simulink model "FinalSim"  (R2022b)
settings: Solver=VariableStepAuto  StartTime=0.0  StopTime=10  RelTol=1e-3
libraries: eeGeneralControl x3
(part 1 of 7)
settings Model: Creator=Dhruv  LastModifiedBy=Dhruv

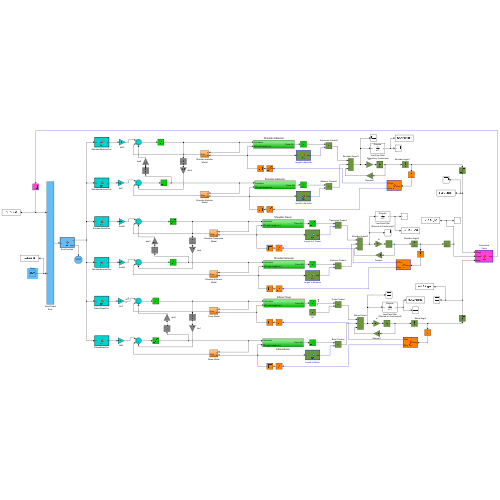
[thumbnail: Simulink's stored preview of the top-level diagram]
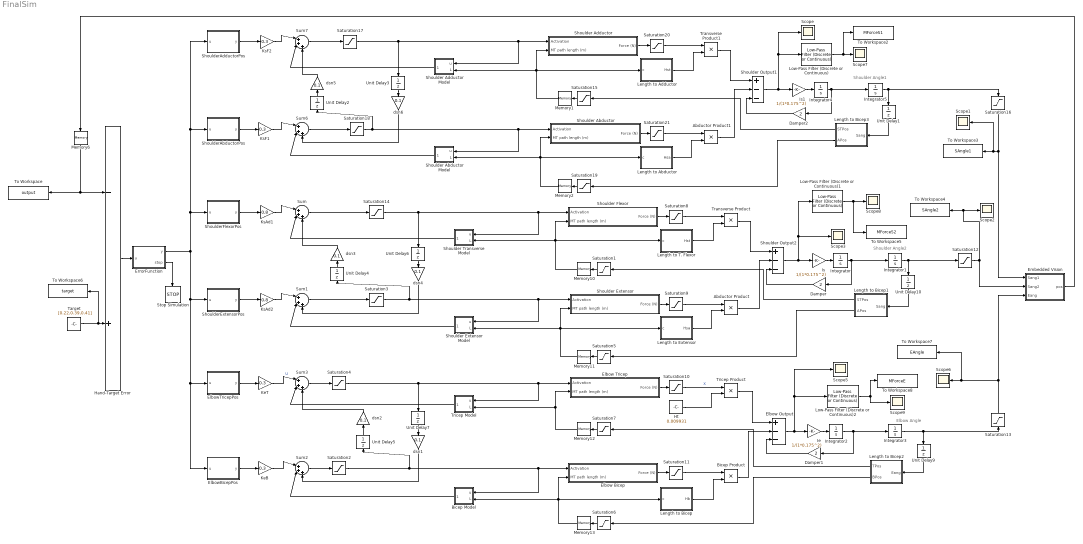
== system FinalSim ==
  note: Shoulder Angle2
  note: Elbow Angle
  note: Shoulder Angle1
  Abductor Product : Product  RndMeth=Zero
  Abductor Product1 : Product  RndMeth=Zero
  Bicep Model : Subsystem
  Bicep Product : Product  RndMeth=Zero
  Damper : Gain  Gain=2
  Damper1 : Gain  Gain=2
  Damper2 : Gain  Gain=2
  Elbow Bicep : Subsystem
  Elbow Output : Sum  Inputs=+--
  Elbow Tricep : Subsystem
  "ElbowBicepPos " : MATLAB Function  TreatAsAtomicUnit=on
  "ElbowTricepPos " : MATLAB Function  TreatAsAtomicUnit=on
  Embedded Vision : MATLAB Function  TreatAsAtomicUnit=on
  ErrorFunction : MATLAB Function  TreatAsAtomicUnit=on
  Hand-Target Error : Sum  Inputs=-+
  Ht : Constant  Value=0.009931  VectorParams1D=off
  Ie : Gain  Gain=1/(1*0.175^2)
  Integrator : Integrator  ZeroCross=off
  Integrator1 : Integrator  InitialCondition=0.5673
  Integrator2 : Integrator  ZeroCross=off
  Integrator3 : Integrator  InitialCondition=0.2362
  Integrator4 : Integrator  ZeroCross=off
  Integrator5 : Integrator  InitialCondition=0.838
  Is : Gain  Gain=1/(1*0.175^2)
  Is1 : Gain  Gain=1/(1*0.175^2)
  KeB : Gain  Gain=0.3
  KeT : Gain  Gain=0.3
  KsAd1 : Gain  Gain=0.8
  KsAd2 : Gain  Gain=0.8
  KsF1 : Gain  Gain=0.3
  KsF2 : Gain  Gain=0.3
  Length to Abductor : MATLAB Function  TreatAsAtomicUnit=on
  Length to Adductor : MATLAB Function  TreatAsAtomicUnit=on
  Length to Bicep : MATLAB Function  TreatAsAtomicUnit=on
  Length to Bicep1 : MATLAB Function  TreatAsAtomicUnit=on
  Length to Bicep2 : MATLAB Function  TreatAsAtomicUnit=on
  Length to Bicep3 : MATLAB Function  TreatAsAtomicUnit=on
  Length to Extensor : MATLAB Function  TreatAsAtomicUnit=on
  Length to T. Flexor : MATLAB Function  TreatAsAtomicUnit=on
  Low-Pass Filter (Discrete or Continuous) : eeGeneralControl/Low-Pass Filter (Discrete or Continuous)  K=1  T=1  B=inf  A=-inf  init_option=Inherited from block input  x0=0  Ts=-1
  Low-Pass Filter (Discrete or Continuous)1 : eeGeneralControl/Low-Pass Filter (Discrete or Continuous)  K=1  T=1  B=inf  A=-inf  init_option=Inherited from block input  x0=0  Ts=-1
  Low-Pass Filter (Discrete or Continuous)2 : eeGeneralControl/Low-Pass Filter (Discrete or Continuous)  K=1  T=1  B=inf  A=-inf  init_option=Inherited from block input  x0=0  Ts=-1
  Memory1 : Memory  InitialCondition=0.08165  InheritSampleTime=on
  Memory10 : Memory  InitialCondition=0.08943  InheritSampleTime=on
  Memory11 : Memory  InitialCondition=0.06893  InheritSampleTime=on
  Memory12 : Memory  InitialCondition=0.1729  InheritSampleTime=on
  Memory13 : Memory  InitialCondition=0.1076  InheritSampleTime=on
  Memory2 : Memory  InitialCondition=0.06454  InheritSampleTime=on
  Memory6 : Memory  InitialCondition=[0.16960,0.1895620 , 0.2307203]  InheritSampleTime=on
  Saturation1 : Saturate  UpperLimit=0.095  LowerLimit=0.068  LinearizeAsGain=off
  Saturation{8..11,20..21} (6 alike) : Saturate  UpperLimit=200  LowerLimit=0  LinearizeAsGain=off
  Saturation12 : Saturate  UpperLimit=3.14159  LowerLimit=-1.0472  LinearizeAsGain=off
  Saturation13 : Saturate  UpperLimit=2.61799  LowerLimit=0  LinearizeAsGain=off
  Saturation{2..4,14,17..18} (6 alike) : Saturate  UpperLimit=1  LowerLimit=0  LinearizeAsGain=off
  Saturation15 : Saturate  UpperLimit=0.095  LowerLimit=0.068  LinearizeAsGain=off
  Saturation16 : Saturate  UpperLimit=2.61799  LowerLimit=-0.872665  LinearizeAsGain=off
  Saturation19 : Saturate  UpperLimit=0.075  LowerLimit=0.057  LinearizeAsGain=off
  Saturation5 : Saturate  UpperLimit=0.075  LowerLimit=0.057  LinearizeAsGain=off
  Saturation6 : Saturate  UpperLimit=0.15  LowerLimit=0.1  LinearizeAsGain=off  RndMeth=Nearest
  Saturation7 : Saturate  UpperLimit=0.17  LowerLimit=0.1  LinearizeAsGain=off
  Scope{,1..3,5..9} (9 alike) : Scope
  Shoulder Abductor : Subsystem
  Shoulder Abductor Model : Subsystem
  Shoulder Adductor : Subsystem
  Shoulder Adductor Model : Subsystem
  Shoulder Extensor : Subsystem
  Shoulder Extensor Model : Subsystem
  Shoulder Flexor : Subsystem
  Shoulder Output1 : Sum  Inputs=+--
  Shoulder Output2 : Sum  Inputs=+--
  Shoulder Transverse Model : Subsystem
  "ShoulderAbductorPos " : MATLAB Function  TreatAsAtomicUnit=on
  "ShoulderAdductorPos " : MATLAB Function  TreatAsAtomicUnit=on
  "ShoulderExtensorPos " : MATLAB Function  TreatAsAtomicUnit=on
  "ShoulderFlexorPos " : MATLAB Function  TreatAsAtomicUnit=on
  Stop Simulation : Stop
  Sum{,1..3,6..7} (6 alike) : Sum  Inputs=|+++  OutMin=[-10]  OutMax=[10]  SampleTime=0.04
  Target : Constant  Value=[0.22,0.39,0.41]  VectorParams1D=off
  To Workspace : ToWorkspace  VariableName=output  SaveFormat=Timeseries  SampleTime=-1
  To Workspace2 : ToWorkspace  VariableName=MForceS1  SaveFormat=Timeseries  SampleTime=-1
  To Workspace3 : ToWorkspace  VariableName=SAngle1  SaveFormat=Timeseries  SampleTime=-1
  To Workspace4 : ToWorkspace  VariableName=SAngle2  SaveFormat=Timeseries  SampleTime=-1
  To Workspace5 : ToWorkspace  VariableName=MForceS2  SaveFormat=Timeseries  SampleTime=-1
  To Workspace6 : ToWorkspace  VariableName=target  SaveFormat=Timeseries  SampleTime=-1
  To Workspace7 : ToWorkspace  VariableName=EAngle  SaveFormat=Timeseries  SampleTime=-1
  To Workspace8 : ToWorkspace  VariableName=MForceE  SaveFormat=Timeseries  SampleTime=-1
  Transverse Product : Product  RndMeth=Zero
  Transverse Product1 : Product  RndMeth=Zero
  Tricep Model : Subsystem
  Tricep Product : Product  RndMeth=Zero
  Unit Delay{1..7,9..10} (9 alike) : UnitDelay  SampleTime=-1
  dsn{1..6} (6 alike) : Gain  Gain=0.1
  wires:
  Shoulder Transverse Model/1(Fom) -> Sum/2
  Is/1 -> Integrator/1
  Ie/1 -> Integrator2/1
  Memory10/1 -> Shoulder Flexor/2(MT path length (m)), Length to T. Flexor/1(c), Shoulder Transverse Model/2(L)
  Saturation13/1 -> Embedded Vision/3(Eang), To Workspace7/1, Scope6/1
  Unit Delay5/1 -> dsn2/1
  Integrator1/1 -> Unit Delay10/1, Saturation12/1
  Saturation3/1 -> Unit Delay4/1, Shoulder Extensor Model/1(u), Shoulder Extensor/1(Activation)
  Damper/1 -> Shoulder Output2/3
  dsn3/1 -> Sum/3
  Saturation11/1 -> Bicep Product/1
  Saturation6/1 -> Memory13/1
  Target/1 -> To Workspace6/1, Hand-Target Error/2
  Damper1/1 -> Elbow Output/3
  Saturation8/1 -> Transverse Product/1
  Saturation10/1 -> Tricep Product/1  "X"
  Saturation9/1 -> Abductor Product/1
  Elbow Tricep/1(Force (N)) -> Saturation10/1
  Memory11/1 -> Shoulder Extensor/2(MT path length (m)), Length to Extensor/1(c), Shoulder Extensor Model/2(L)
  Memory13/1 -> Length to Bicep/1(c), Bicep Model/2(L), Elbow Bicep/2(MT path length (m))
  Integrator/1 -> Damper/1, Integrator1/1
  Saturation12/1 -> To Workspace4/1, Scope2/1, Embedded Vision/2(Sang2)
  Transverse Product/1 -> Shoulder Output2/1
  Abductor Product/1 -> Shoulder Output2/2
  Length to T. Flexor/1(Hst) -> Transverse Product/2
  Length to Extensor/1(Hsa) -> Abductor Product/2
  Memory12/1 -> Elbow Tricep/2(MT path length (m)), Tricep Model/2(L)
  Saturation7/1 -> Memory12/1
  Shoulder Flexor/1(Force (N)) -> Saturation8/1
  Tricep Product/1 -> Elbow Output/1
  Ht/1 -> Tricep Product/2
  Elbow Bicep/1(Force (N)) -> Saturation11/1
  Integrator3/1 -> Saturation13/1, Unit Delay9/1
  Unit Delay7/1 -> dsn1/1
  Integrator2/1 -> Damper1/1, Integrator3/1
  Saturation1/1 -> Memory10/1
  Length to Bicep/1(Hb) -> Bicep Product/2
  dsn1/1 -> Sum2/3
  Memory6/1 -> To Workspace/1, Hand-Target Error/1
  Unit Delay4/1 -> dsn3/1
  Unit Delay6/1 -> dsn4/1
  Shoulder Extensor/1(Force (N)) -> Saturation9/1
  Saturation5/1 -> Memory11/1
  Sum/1 -> Saturation14/1
  Bicep Product/1 -> Elbow Output/2
  Shoulder Abductor/1(Force (N)) -> Saturation21/1
  Unit Delay3/1 -> dsn6/1
  Saturation19/1 -> Memory2/1
  Unit Delay2/1 -> dsn5/1
  Saturation15/1 -> Memory1/1
  Shoulder Output1/1 -> Is1/1, Scope/1, Low-Pass Filter (Discrete or Continuous)/1
  Shoulder Adductor/1(Force (N)) -> Saturation20/1
  Abductor Product1/1 -> Shoulder Output1/2
  Saturation16/1 -> Embedded Vision/1(Sang1), Scope1/1, To Workspace3/1
  Integrator4/1 -> Damper2/1, Integrator5/1
  Length to Abductor/1(Hsa) -> Abductor Product1/2
  Damper2/1 -> Shoulder Output1/3
  Memory2/1 -> Shoulder Abductor/2(MT path length (m)), Length to Abductor/1(c), Shoulder Abductor Model/2(L)
  Length to Adductor/1(Hst) -> Transverse Product1/2
  Is1/1 -> Integrator4/1
  Transverse Product1/1 -> Shoulder Output1/1
  Memory1/1 -> Shoulder Adductor/2(MT path length (m)), Length to Adductor/1(c), Shoulder Adductor Model/2(L)
  Saturation20/1 -> Transverse Product1/1
  Saturation21/1 -> Abductor Product1/1
  Hand-Target Error/1 -> ErrorFunction/1(u)
  "ShoulderFlexorPos "/1(y) -> KsAd1/1
  "ShoulderExtensorPos "/1(y) -> KsAd2/1
  "ElbowTricepPos "/1(y) -> KeT/1
  "ElbowBicepPos "/1(y) -> KeB/1
  "ShoulderAbductorPos "/1(y) -> KsF1/1
  "ShoulderAdductorPos "/1(y) -> KsF2/1
  ErrorFunction/2(stop) -> Stop Simulation/1
  Embedded Vision/1(pos) -> Memory6/1
  Integrator5/1 -> Saturation16/1, Unit Delay1/1
  Unit Delay9/1 -> Length to Bicep2/1(Eang)
  Length to Bicep2/1(TPos) -> Saturation7/1
  Length to Bicep2/2(BPos) -> Saturation6/1
  Sum3/1 -> Saturation4/1
  dsn2/1 -> Sum3/3
  Tricep Model/1(Fom) -> Sum3/2
  dsn4/1 -> Sum1/3
  Shoulder Extensor Model/1(Fom) -> Sum1/2
  Sum2/1 -> Saturation2/1
  Bicep Model/1(Fom) -> Sum2/2
  Sum6/1 -> Saturation18/1
  Sum7/1 -> Saturation17/1
  dsn5/1 -> Sum7/3
  Shoulder Adductor Model/1(Fom) -> Sum7/2
  dsn6/1 -> Sum6/3
  Shoulder Abductor Model/1(Fom) -> Sum6/2
  Low-Pass Filter (Discrete or Continuous)/1 -> Scope7/1, To Workspace2/1
  Low-Pass Filter (Discrete or Continuous)1/1 -> To Workspace5/1, Scope8/1
  Shoulder Output2/1 -> Low-Pass Filter (Discrete or Continuous)1/1, Scope3/1, Is/1
  Low-Pass Filter (Discrete or Continuous)2/1 -> Scope9/1, To Workspace8/1
  Elbow Output/1 -> Scope5/1, Low-Pass Filter (Discrete or Continuous)2/1, Ie/1
  Unit Delay1/1 -> Length to Bicep3/1(Sang)
  Unit Delay10/1 -> Length to Bicep1/1(Sang)
  Length to Bicep1/2(APos) -> Saturation5/1
  Length to Bicep1/1(STPos) -> Saturation1/1
  ErrorFunction/1(y) -> "ShoulderAdductorPos "/1(u), "ShoulderAbductorPos "/1(u), "ShoulderFlexorPos "/1(u), "ElbowBicepPos "/1(u), "ElbowTricepPos "/1(u), "ShoulderExtensorPos "/1(u)
  Length to Bicep3/2(APos) -> Saturation19/1
  Length to Bicep3/1(STPos) -> Saturation15/1
  KsAd1/1 -> Sum/1
  KsAd2/1 -> Sum1/1
  KeB/1 -> Sum2/1
  KeT/1 -> Sum3/1  "U"
  Saturation4/1 -> Unit Delay7/1, Tricep Model/1(u), Elbow Tricep/1(Activation)
  Saturation2/1 -> Unit Delay5/1, Bicep Model/1(u), Elbow Bicep/1(Activation)
  Sum1/1 -> Saturation3/1
  Saturation14/1 -> Unit Delay6/1, Shoulder Transverse Model/1(u), Shoulder Flexor/1(Activation)
  Saturation18/1 -> Shoulder Abductor Model/1(u), Shoulder Abductor/1(Activation), Unit Delay2/1
  Saturation17/1 -> Unit Delay3/1, Shoulder Adductor Model/1(u), Shoulder Adductor/1(Activation)
  KsF2/1 -> Sum7/1
  KsF1/1 -> Sum6/1

== system FinalSim/Bicep Model ==
  u : Inport
  L : Inport  Port=2
  Bicep Group1 : Subsystem
  Saturation18 : Saturate  UpperLimit=200  LowerLimit=0  LinearizeAsGain=off
  dbi : Gain  Gain=1/1000
  Fom : Outport
  wires:
  dbi/1 -> Fom/1
  Bicep Group1/1(Force (N)) -> Saturation18/1
  Saturation18/1 -> dbi/1
  u/1 -> Bicep Group1/1(Activation)
  L/1 -> Bicep Group1/2(MT path length (m))

== system FinalSim/Elbow Bicep ==
  Activation : Inport
  MT path length (m) : Inport  Port=2
  Convert m to cm : Gain  Gain=100  SaturateOnIntegerOverflow=on  OutDataTypeStr=Inherit: Same as input  ParamDataTypeStr=Inherit: Same as input
  Recruitment : Subsystem
  fascicles (CE & PE) : Subsystem
  muscle mass : Subsystem
  series elastic element : Subsystem
  Force (N) : Outport
  wires:
  MT path length (m)/1 -> Convert m to cm/1
  series elastic element/1(Fse (N)) -> muscle mass/2(Fse (N)), Force (N)/1
  fascicles (CE & PE)/1(Force (N)) -> muscle mass/1(Fce (N))
  muscle mass/2(Lce (L0)) -> fascicles (CE & PE)/2(Length (L0)), series elastic element/2(Lce (L0))
  muscle mass/1(Vce (L0/s)) -> fascicles (CE & PE)/3(Velocity (L0/s))
  Recruitment/1(Frequencies (f0.5)) -> fascicles (CE & PE)/1(Frequencies (f0.5))
  Convert m to cm/1 -> series elastic element/1(Path (cm)), muscle mass/3(Path length [for init] (cm))
  Activation/1 -> Recruitment/1(Activation)

== system FinalSim/Elbow Tricep ==
  Activation : Inport
  MT path length (m) : Inport  Port=2
  Convert m to cm : Gain  Gain=100  SaturateOnIntegerOverflow=on  OutDataTypeStr=Inherit: Same as input  ParamDataTypeStr=Inherit: Same as input
  Recruitment : Subsystem
  fascicles (CE & PE) : Subsystem
  muscle mass : Subsystem
  series elastic element : Subsystem
  Force (N) : Outport
  wires:
  MT path length (m)/1 -> Convert m to cm/1
  series elastic element/1(Fse (N)) -> muscle mass/2(Fse (N)), Force (N)/1
  fascicles (CE & PE)/1(Force (N)) -> muscle mass/1(Fce (N))
  muscle mass/2(Lce (L0)) -> series elastic element/2(Lce (L0)), fascicles (CE & PE)/2(Length (L0))
  muscle mass/1(Vce (L0/s)) -> fascicles (CE & PE)/3(Velocity (L0/s))
  Recruitment/1(Frequencies (f0.5)) -> fascicles (CE & PE)/1(Frequencies (f0.5))
  Convert m to cm/1 -> series elastic element/1(Path (cm)), muscle mass/3(Path length [for init] (cm))
  Activation/1 -> Recruitment/1(Activation)

== system FinalSim/Shoulder Abductor ==
  Activation : Inport
  MT path length (m) : Inport  Port=2
  Convert m to cm : Gain  Gain=100  SaturateOnIntegerOverflow=on  OutDataTypeStr=Inherit: Same as input  ParamDataTypeStr=Inherit: Same as input
  Recruitment : Subsystem
  fascicles (CE & PE) : Subsystem
  muscle mass : Subsystem
  series elastic element : Subsystem
  Force (N) : Outport
  wires:
  MT path length (m)/1 -> Convert m to cm/1
  series elastic element/1(Fse (N)) -> muscle mass/2(Fse (N)), Force (N)/1
  fascicles (CE & PE)/1(Force (N)) -> muscle mass/1(Fce (N))
  muscle mass/2(Lce (L0)) -> series elastic element/2(Lce (L0)), fascicles (CE & PE)/2(Length (L0))
  muscle mass/1(Vce (L0/s)) -> fascicles (CE & PE)/3(Velocity (L0/s))
  Recruitment/1(Frequencies (f0.5)) -> fascicles (CE & PE)/1(Frequencies (f0.5))
  Convert m to cm/1 -> series elastic element/1(Path (cm)), muscle mass/3(Path length [for init] (cm))
  Activation/1 -> Recruitment/1(Activation)

== system FinalSim/Shoulder Abductor Model ==
  u : Inport
  L : Inport  Port=2
  Saturation15 : Saturate  UpperLimit=200  LowerLimit=0  LinearizeAsGain=off
  Shoulder Abductors1 : Subsystem
  dsa : Gain  Gain=1/1000
  Fom : Outport
  wires:
  dsa/1 -> Fom/1
  Shoulder Abductors1/1(Force (N)) -> Saturation15/1
  Saturation15/1 -> dsa/1
  u/1 -> Shoulder Abductors1/1(Activation)
  L/1 -> Shoulder Abductors1/2(MT path length (m))

== system FinalSim/Shoulder Adductor ==
  Activation : Inport
  MT path length (m) : Inport  Port=2
  Convert m to cm : Gain  Gain=100  SaturateOnIntegerOverflow=on  OutDataTypeStr=Inherit: Same as input  ParamDataTypeStr=Inherit: Same as input
  Recruitment : Subsystem
  fascicles (CE & PE) : Subsystem
  muscle mass : Subsystem
  series elastic element : Subsystem
  Force (N) : Outport
  wires:
  MT path length (m)/1 -> Convert m to cm/1
  series elastic element/1(Fse (N)) -> muscle mass/2(Fse (N)), Force (N)/1
  fascicles (CE & PE)/1(Force (N)) -> muscle mass/1(Fce (N))
  muscle mass/2(Lce (L0)) -> series elastic element/2(Lce (L0)), fascicles (CE & PE)/2(Length (L0))
  muscle mass/1(Vce (L0/s)) -> fascicles (CE & PE)/3(Velocity (L0/s))
  Recruitment/1(Frequencies (f0.5)) -> fascicles (CE & PE)/1(Frequencies (f0.5))
  Convert m to cm/1 -> series elastic element/1(Path (cm)), muscle mass/3(Path length [for init] (cm))
  Activation/1 -> Recruitment/1(Activation)

== system FinalSim/Shoulder Adductor Model ==
  u : Inport
  L : Inport  Port=2
  Saturation16 : Saturate  UpperLimit=200  LowerLimit=0  LinearizeAsGain=off
  Shoulder Transverse Flexors1 : Subsystem
  dst : Gain  Gain=1/1000
  Fom : Outport
  wires:
  dst/1 -> Fom/1
  Shoulder Transverse Flexors1/1(Force (N)) -> Saturation16/1
  Saturation16/1 -> dst/1
  u/1 -> Shoulder Transverse Flexors1/1(Activation)
  L/1 -> Shoulder Transverse Flexors1/2(MT path length (m))

== system FinalSim/Shoulder Extensor ==
  Activation : Inport
  MT path length (m) : Inport  Port=2
  Convert m to cm : Gain  Gain=100  SaturateOnIntegerOverflow=on  OutDataTypeStr=Inherit: Same as input  ParamDataTypeStr=Inherit: Same as input
  Recruitment : Subsystem
  fascicles (CE & PE) : Subsystem
  muscle mass : Subsystem
  series elastic element : Subsystem
  Force (N) : Outport
  wires:
  MT path length (m)/1 -> Convert m to cm/1
  series elastic element/1(Fse (N)) -> muscle mass/2(Fse (N)), Force (N)/1
  fascicles (CE & PE)/1(Force (N)) -> muscle mass/1(Fce (N))
  muscle mass/2(Lce (L0)) -> series elastic element/2(Lce (L0)), fascicles (CE & PE)/2(Length (L0))
  muscle mass/1(Vce (L0/s)) -> fascicles (CE & PE)/3(Velocity (L0/s))
  Recruitment/1(Frequencies (f0.5)) -> fascicles (CE & PE)/1(Frequencies (f0.5))
  Convert m to cm/1 -> series elastic element/1(Path (cm)), muscle mass/3(Path length [for init] (cm))
  Activation/1 -> Recruitment/1(Activation)

== system FinalSim/Shoulder Extensor Model ==
  u : Inport
  L : Inport  Port=2
  Saturation15 : Saturate  UpperLimit=200  LowerLimit=0  LinearizeAsGain=off
  Shoulder Abductors1 : Subsystem
  dsa : Gain  Gain=1/1000
  Fom : Outport
  wires:
  dsa/1 -> Fom/1
  Shoulder Abductors1/1(Force (N)) -> Saturation15/1
  Saturation15/1 -> dsa/1
  u/1 -> Shoulder Abductors1/1(Activation)
  L/1 -> Shoulder Abductors1/2(MT path length (m))

== system FinalSim/Shoulder Flexor ==
  Activation : Inport
  MT path length (m) : Inport  Port=2
  Convert m to cm : Gain  Gain=100  SaturateOnIntegerOverflow=on  OutDataTypeStr=Inherit: Same as input  ParamDataTypeStr=Inherit: Same as input
  Recruitment : Subsystem
  fascicles (CE & PE) : Subsystem
  muscle mass : Subsystem
  series elastic element : Subsystem
  Force (N) : Outport
  wires:
  MT path length (m)/1 -> Convert m to cm/1
  series elastic element/1(Fse (N)) -> muscle mass/2(Fse (N)), Force (N)/1
  fascicles (CE & PE)/1(Force (N)) -> muscle mass/1(Fce (N))
  muscle mass/2(Lce (L0)) -> series elastic element/2(Lce (L0)), fascicles (CE & PE)/2(Length (L0))
  muscle mass/1(Vce (L0/s)) -> fascicles (CE & PE)/3(Velocity (L0/s))
  Recruitment/1(Frequencies (f0.5)) -> fascicles (CE & PE)/1(Frequencies (f0.5))
  Convert m to cm/1 -> series elastic element/1(Path (cm)), muscle mass/3(Path length [for init] (cm))
  Activation/1 -> Recruitment/1(Activation)

== system FinalSim/Shoulder Transverse Model ==
  u : Inport
  L : Inport  Port=2
  Saturation16 : Saturate  UpperLimit=200  LowerLimit=0  LinearizeAsGain=off
  Shoulder Transverse Flexors1 : Subsystem
  dst : Gain  Gain=1/1000
  Fom : Outport
  wires:
  dst/1 -> Fom/1
  Shoulder Transverse Flexors1/1(Force (N)) -> Saturation16/1
  Saturation16/1 -> dst/1
  u/1 -> Shoulder Transverse Flexors1/1(Activation)
  L/1 -> Shoulder Transverse Flexors1/2(MT path length (m))

== system FinalSim/Tricep Model ==
  u : Inport
  L : Inport  Port=2
  Saturation17 : Saturate  UpperLimit=200  LowerLimit=0  LinearizeAsGain=off
  Tricep Group : Subsystem
  dtr : Gain  Gain=1/1000  OutMin=[-10]  OutMax=[10]
  Fom : Outport
  wires:
  dtr/1 -> Fom/1
  Tricep Group/1(Force (N)) -> Saturation17/1
  Saturation17/1 -> dtr/1
  u/1 -> Tricep Group/1(Activation)
  L/1 -> Tricep Group/2(MT path length (m))

== system FinalSim/Bicep Model/Bicep Group1 ==
  Activation : Inport
  MT path length (m) : Inport  Port=2
  Convert m to cm : Gain  Gain=100  SaturateOnIntegerOverflow=on  OutDataTypeStr=Inherit: Same as input  ParamDataTypeStr=Inherit: Same as input
  Recruitment : Subsystem
  fascicles (CE & PE) : Subsystem
  muscle mass : Subsystem
  series elastic element : Subsystem
  Force (N) : Outport
  wires:
  MT path length (m)/1 -> Convert m to cm/1
  series elastic element/1(Fse (N)) -> muscle mass/2(Fse (N)), Force (N)/1
  fascicles (CE & PE)/1(Force (N)) -> muscle mass/1(Fce (N))
  muscle mass/2(Lce (L0)) -> series elastic element/2(Lce (L0)), fascicles (CE & PE)/2(Length (L0))
  muscle mass/1(Vce (L0/s)) -> fascicles (CE & PE)/3(Velocity (L0/s))
  Recruitment/1(Frequencies (f0.5)) -> fascicles (CE & PE)/1(Frequencies (f0.5))
  Convert m to cm/1 -> series elastic element/1(Path (cm)), muscle mass/3(Path length [for init] (cm))
  Activation/1 -> Recruitment/1(Activation)

== system FinalSim/Elbow Bicep/Recruitment ==
  Activation : Inport
  Mux all F Units : Mux  Inputs=3
  Mux all S Units : Mux  Inputs=2
  Mux all Units : Mux  Inputs=2
  Type F Motor Unit 1 : Subsystem
  Type F Motor Unit 2 : Subsystem
  Type F Motor Unit 3 : Subsystem
  Type S Motor Unit 1 : Subsystem
  Type S Motor Unit 2 : Subsystem
  Frequencies (f0.5) : Outport
  wires:
  Activation/1 -> Type S Motor Unit 1/1(Activation), Type S Motor Unit 2/1(Activation), Type F Motor Unit 1/1(Activation), Type F Motor Unit 2/1(Activation), Type F Motor Unit 3/1(Activation)
  Type S Motor Unit 1/1(Frequency (f0.5)) -> Mux all S Units/1
  Type S Motor Unit 2/1(Frequency (f0.5)) -> Mux all S Units/2
  Mux all S Units/1 -> Mux all Units/1
  Type F Motor Unit 1/1(Frequency (f0.5)) -> Mux all F Units/1
  Type F Motor Unit 2/1(Frequency (f0.5)) -> Mux all F Units/2
  Type F Motor Unit 3/1(Frequency (f0.5)) -> Mux all F Units/3
  Mux all F Units/1 -> Mux all Units/2
  Mux all Units/1 -> Frequencies (f0.5)/1

== system FinalSim/Elbow Bicep/fascicles (CE & PE) ==
  Frequencies (f0.5) : Inport
  Length (L0) : Inport  Port=2
  Velocity (L0/s) : Inport  Port=3
  Convert F0 to N : Gain  Gain=305.7857  SaturateOnIntegerOverflow=on  OutDataTypeStr=Inherit: Same as input  ParamDataTypeStr=Inherit: Same as input
  Demux all Units : Demux  Outputs="[2  3]"
      settings: DisplayOption=none
  Force>0 : MinMax  Function=max  Inputs=2  InputSameDT=on  SaturateOnIntegerOverflow=on
  Fpe1 : Fcn  Expr=0.01*u(1)+23*0.046*log(exp((u(2)/1.6139-1.17)/0.046)+1)
  Fpe2 : Fcn  Expr=-0.02*(exp(-21.0375*(u-0.70222))-1)
  Min : MinMax  Inputs=2  InputSameDT=on  SaturateOnIntegerOverflow=on
  Sum Forces (F0) : Sum  Inputs=2  InputSameDT=on  SaturateOnIntegerOverflow=on  OutDataTypeStr=Inherit: Same as first input
  Sum all Units (F0) : Sum  InputSameDT=on  SaturateOnIntegerOverflow=on  OutDataTypeStr=Inherit: Same as first input
  Type F Motor Units : Subsystem
  Type S Motor Units : Subsystem
  V,L : Mux  Inputs=2
  zero : Constant  Value=0
  zero2 : Constant  Value=0
  Force (N) : Outport
  wires:
  Demux all Units/1 -> Type S Motor Units/1(fenv)
  V,L/1 -> Type S Motor Units/2(V,L), Type F Motor Units/2(V,L), Fpe1/1
  Min/1 -> Type S Motor Units/3(Fpe2), Type F Motor Units/3(Fpe2)
  Type S Motor Units/1(F (Fo)) -> Sum all Units (F0)/1
  Demux all Units/2 -> Type F Motor Units/1(fenv)
  Type F Motor Units/1(F (Fo)) -> Sum all Units (F0)/2
  Length (L0)/1 -> Fpe2/1, V,L/2
  Velocity (L0/s)/1 -> V,L/1
  Fpe2/1 -> Min/1
  zero2/1 -> Min/2
  Frequencies (f0.5)/1 -> Demux all Units/1
  Convert F0 to N/1 -> Force>0/1
  zero/1 -> Force>0/2
  Force>0/1 -> Force (N)/1
  Fpe1/1 -> Sum Forces (F0)/1
  Sum all Units (F0)/1 -> Sum Forces (F0)/2
  Sum Forces (F0)/1 -> Convert F0 to N/1

== system FinalSim/Elbow Bicep/muscle mass ==
  Fce (N) : Inport
  Fse (N) : Inport  Port=2
  Path length [for init] (cm) : Inport  Port=3
  Acc to Vel : Integrator
  Force/Mass=Accel : Gain  Gain=1/0.035675  SaturateOnIntegerOverflow=on  OutDataTypeStr=Inherit: Same as input  ParamDataTypeStr=Inherit: Same as input
  Ftotal : Sum  Inputs=-+  InputSameDT=on  SaturateOnIntegerOverflow=on  OutDataTypeStr=Inherit: Same as first input
  Normalize to L0 : Gain  Gain=1/0.07  SaturateOnIntegerOverflow=on  OutDataTypeStr=Inherit: Same as input  ParamDataTypeStr=Inherit: Same as input
  Normalize to L0/s : Gain  Gain=1/0.07  SaturateOnIntegerOverflow=on  OutDataTypeStr=Inherit: Same as input  ParamDataTypeStr=Inherit: Same as input
  Path to init muscle mass position (m) : Fcn  Expr=(u-5.2966)/105.6073
  Vel to Pos : Integrator  InitialConditionSource=external
  Vce (L0/s) : Outport
  Lce (L0) : Outport  Port=2
  wires:
  Ftotal/1 -> Force/Mass=Accel/1
  Force/Mass=Accel/1 -> Acc to Vel/1
  Acc to Vel/1 -> Vel to Pos/1, Normalize to L0/s/1
  Path length [for init] (cm)/1 -> Path to init muscle mass position (m)/1
  Path to init muscle mass position (m)/1 -> Vel to Pos/2
  Vel to Pos/1 -> Normalize to L0/1
  Fce (N)/1 -> Ftotal/1
  Normalize to L0/1 -> Lce (L0)/1
  Fse (N)/1 -> Ftotal/2
  Normalize to L0/s/1 -> Vce (L0/s)/1

== system FinalSim/Elbow Bicep/series elastic element ==
  Path (cm) : Inport
  Lce (L0) : Inport  Port=2
  Convert Lce to Lse : Sum  Inputs=+-  InputSameDT=on  SaturateOnIntegerOverflow=on  OutDataTypeStr=Inherit: Same as first input
  Convert to N : Gain  Gain=305.7857  SaturateOnIntegerOverflow=on  OutDataTypeStr=Inherit: Same as input  ParamDataTypeStr=Inherit: Same as input
  Convert to cm : Gain  Gain=7  SaturateOnIntegerOverflow=on  OutDataTypeStr=Inherit: Same as input  ParamDataTypeStr=Inherit: Same as input
  Fse : Fcn  Expr=27.8*0.0047*log(exp((u(1)-0.964)/0.0047)+1)
  Normalize to L0T : Gain  Gain=1/6.2  SaturateOnIntegerOverflow=on  OutDataTypeStr=Inherit: Same as input  ParamDataTypeStr=Inherit: Same as input
  Fse (N) : Outport
  wires:
  Fse/1 -> Convert to N/1
  Normalize to L0T/1 -> Fse/1
  Convert Lce to Lse/1 -> Normalize to L0T/1
  Convert to N/1 -> Fse (N)/1
  Lce (L0)/1 -> Convert to cm/1
  Convert to cm/1 -> Convert Lce to Lse/2
  Path (cm)/1 -> Convert Lce to Lse/1

== system FinalSim/Elbow Tricep/Recruitment ==
  Activation : Inport
  Mux all F Units : Mux  Inputs=3
  Mux all S Units : Mux  Inputs=2
  Mux all Units : Mux  Inputs=2
  Type F Motor Unit 1 : Subsystem
  Type F Motor Unit 2 : Subsystem
  Type F Motor Unit 3 : Subsystem
  Type S Motor Unit 1 : Subsystem
  Type S Motor Unit 2 : Subsystem
  Frequencies (f0.5) : Outport
  wires:
  Activation/1 -> Type S Motor Unit 1/1(Activation), Type S Motor Unit 2/1(Activation), Type F Motor Unit 1/1(Activation), Type F Motor Unit 2/1(Activation), Type F Motor Unit 3/1(Activation)
  Type S Motor Unit 1/1(Frequency (f0.5)) -> Mux all S Units/1
  Type S Motor Unit 2/1(Frequency (f0.5)) -> Mux all S Units/2
  Mux all S Units/1 -> Mux all Units/1
  Type F Motor Unit 1/1(Frequency (f0.5)) -> Mux all F Units/1
  Type F Motor Unit 2/1(Frequency (f0.5)) -> Mux all F Units/2
  Type F Motor Unit 3/1(Frequency (f0.5)) -> Mux all F Units/3
  Mux all F Units/1 -> Mux all Units/2
  Mux all Units/1 -> Frequencies (f0.5)/1

== system FinalSim/Elbow Tricep/fascicles (CE & PE) ==
  Frequencies (f0.5) : Inport
  Length (L0) : Inport  Port=2
  Velocity (L0/s) : Inport  Port=3
  Convert F0 to N : Gain  Gain=422.5714  SaturateOnIntegerOverflow=on  OutDataTypeStr=Inherit: Same as input  ParamDataTypeStr=Inherit: Same as input
  Demux all Units : Demux  Outputs="[2  3]"
      settings: DisplayOption=none
  Force>0 : MinMax  Function=max  Inputs=2  InputSameDT=on  SaturateOnIntegerOverflow=on
  Fpe1 : Fcn  Expr=0.01*u(1)+23*0.046*log(exp((u(2)/1.9394-1.17)/0.046)+1)
  Fpe2 : Fcn  Expr=-0.02*(exp(-21.0375*(u-0.70222))-1)
  Min : MinMax  Inputs=2  InputSameDT=on  SaturateOnIntegerOverflow=on
  Sum Forces (F0) : Sum  Inputs=2  InputSameDT=on  SaturateOnIntegerOverflow=on  OutDataTypeStr=Inherit: Same as first input
  Sum all Units (F0) : Sum  InputSameDT=on  SaturateOnIntegerOverflow=on  OutDataTypeStr=Inherit: Same as first input
  Type F Motor Units : Subsystem
  Type S Motor Units : Subsystem
  V,L : Mux  Inputs=2
  zero : Constant  Value=0
  zero2 : Constant  Value=0
  Force (N) : Outport
  wires:
  Demux all Units/1 -> Type S Motor Units/1(fenv)
  V,L/1 -> Type S Motor Units/2(V,L), Type F Motor Units/2(V,L), Fpe1/1
  Min/1 -> Type S Motor Units/3(Fpe2), Type F Motor Units/3(Fpe2)
  Type S Motor Units/1(F (Fo)) -> Sum all Units (F0)/1
  Demux all Units/2 -> Type F Motor Units/1(fenv)
  Type F Motor Units/1(F (Fo)) -> Sum all Units (F0)/2
  Length (L0)/1 -> Fpe2/1, V,L/2
  Velocity (L0/s)/1 -> V,L/1
  Fpe2/1 -> Min/1
  zero2/1 -> Min/2
  Frequencies (f0.5)/1 -> Demux all Units/1
  Convert F0 to N/1 -> Force>0/1
  zero/1 -> Force>0/2
  Force>0/1 -> Force (N)/1
  Fpe1/1 -> Sum Forces (F0)/1
  Sum all Units (F0)/1 -> Sum Forces (F0)/2
  Sum Forces (F0)/1 -> Convert F0 to N/1

== system FinalSim/Elbow Tricep/muscle mass ==
  Fce (N) : Inport
  Fse (N) : Inport  Port=2
  Path length [for init] (cm) : Inport  Port=3
  Acc to Vel : Integrator
  Force/Mass=Accel : Gain  Gain=1/0.0493  SaturateOnIntegerOverflow=on  OutDataTypeStr=Inherit: Same as input  ParamDataTypeStr=Inherit: Same as input
  Ftotal : Sum  Inputs=-+  InputSameDT=on  SaturateOnIntegerOverflow=on  OutDataTypeStr=Inherit: Same as first input
  Normalize to L0 : Gain  Gain=1/0.07  SaturateOnIntegerOverflow=on  OutDataTypeStr=Inherit: Same as input  ParamDataTypeStr=Inherit: Same as input
  Normalize to L0/s : Gain  Gain=1/0.07  SaturateOnIntegerOverflow=on  OutDataTypeStr=Inherit: Same as input  ParamDataTypeStr=Inherit: Same as input
  Path to init muscle mass position (m) : Fcn  Expr=(u-5.4674)/104.8167
  Vel to Pos : Integrator  InitialConditionSource=external
  Vce (L0/s) : Outport
  Lce (L0) : Outport  Port=2
  wires:
  Ftotal/1 -> Force/Mass=Accel/1
  Force/Mass=Accel/1 -> Acc to Vel/1
  Acc to Vel/1 -> Vel to Pos/1, Normalize to L0/s/1
  Path length [for init] (cm)/1 -> Path to init muscle mass position (m)/1
  Path to init muscle mass position (m)/1 -> Vel to Pos/2
  Vel to Pos/1 -> Normalize to L0/1
  Fce (N)/1 -> Ftotal/1
  Normalize to L0/1 -> Lce (L0)/1
  Fse (N)/1 -> Ftotal/2
  Normalize to L0/s/1 -> Vce (L0/s)/1

== system FinalSim/Elbow Tricep/series elastic element ==
  Path (cm) : Inport
  Lce (L0) : Inport  Port=2
  Convert Lce to Lse : Sum  Inputs=+-  InputSameDT=on  SaturateOnIntegerOverflow=on  OutDataTypeStr=Inherit: Same as first input
  Convert to N : Gain  Gain=422.5714  SaturateOnIntegerOverflow=on  OutDataTypeStr=Inherit: Same as input  ParamDataTypeStr=Inherit: Same as input
  Convert to cm : Gain  Gain=7  SaturateOnIntegerOverflow=on  OutDataTypeStr=Inherit: Same as input  ParamDataTypeStr=Inherit: Same as input
  Fse : Fcn  Expr=27.8*0.0047*log(exp((u(1)-0.964)/0.0047)+1)
  Normalize to L0T : Gain  Gain=1/6.4  SaturateOnIntegerOverflow=on  OutDataTypeStr=Inherit: Same as input  ParamDataTypeStr=Inherit: Same as input
  Fse (N) : Outport
  wires:
  Fse/1 -> Convert to N/1
  Normalize to L0T/1 -> Fse/1
  Convert Lce to Lse/1 -> Normalize to L0T/1
  Convert to N/1 -> Fse (N)/1
  Lce (L0)/1 -> Convert to cm/1
  Convert to cm/1 -> Convert Lce to Lse/2
  Path (cm)/1 -> Convert Lce to Lse/1

== system FinalSim/Shoulder Abductor/Recruitment ==
  Activation : Inport
  Mux all F Units : Mux  Inputs=3
  Mux all S Units : Mux  Inputs=2
  Mux all Units : Mux  Inputs=2
  Type F Motor Unit 1 : Subsystem
  Type F Motor Unit 2 : Subsystem
  Type F Motor Unit 3 : Subsystem
  Type S Motor Unit 1 : Subsystem
  Type S Motor Unit 2 : Subsystem
  Frequencies (f0.5) : Outport
  wires:
  Activation/1 -> Type S Motor Unit 1/1(Activation), Type S Motor Unit 2/1(Activation), Type F Motor Unit 1/1(Activation), Type F Motor Unit 2/1(Activation), Type F Motor Unit 3/1(Activation)
  Type S Motor Unit 1/1(Frequency (f0.5)) -> Mux all S Units/1
  Type S Motor Unit 2/1(Frequency (f0.5)) -> Mux all S Units/2
  Mux all S Units/1 -> Mux all Units/1
  Type F Motor Unit 1/1(Frequency (f0.5)) -> Mux all F Units/1
  Type F Motor Unit 2/1(Frequency (f0.5)) -> Mux all F Units/2
  Type F Motor Unit 3/1(Frequency (f0.5)) -> Mux all F Units/3
  Mux all F Units/1 -> Mux all Units/2
  Mux all Units/1 -> Frequencies (f0.5)/1

== system FinalSim/Shoulder Abductor/fascicles (CE & PE) ==
  Frequencies (f0.5) : Inport
  Length (L0) : Inport  Port=2
  Velocity (L0/s) : Inport  Port=3
  Convert F0 to N : Gain  Gain=307.5  SaturateOnIntegerOverflow=on  OutDataTypeStr=Inherit: Same as input  ParamDataTypeStr=Inherit: Same as input
  Demux all Units : Demux  Outputs="[2  3]"
      settings: DisplayOption=none
  Force>0 : MinMax  Function=max  Inputs=2  InputSameDT=on  SaturateOnIntegerOverflow=on
  Fpe1 : Fcn  Expr=0.01*u(1)+23*0.046*log(exp((u(2)/1.4218-1.17)/0.046)+1)
  Fpe2 : Fcn  Expr=-0.02*(exp(-21.0375*(u-0.70222))-1)
  Min : MinMax  Inputs=2  InputSameDT=on  SaturateOnIntegerOverflow=on
  Sum Forces (F0) : Sum  Inputs=2  InputSameDT=on  SaturateOnIntegerOverflow=on  OutDataTypeStr=Inherit: Same as first input
  Sum all Units (F0) : Sum  InputSameDT=on  SaturateOnIntegerOverflow=on  OutDataTypeStr=Inherit: Same as first input
  Type F Motor Units : Subsystem
  Type S Motor Units : Subsystem
  V,L : Mux  Inputs=2
  zero : Constant  Value=0
  zero2 : Constant  Value=0
  Force (N) : Outport
  wires:
  Demux all Units/1 -> Type S Motor Units/1(fenv)
  V,L/1 -> Type S Motor Units/2(V,L), Type F Motor Units/2(V,L), Fpe1/1
  Min/1 -> Type S Motor Units/3(Fpe2), Type F Motor Units/3(Fpe2)
  Type S Motor Units/1(F (Fo)) -> Sum all Units (F0)/1
  Demux all Units/2 -> Type F Motor Units/1(fenv)
  Type F Motor Units/1(F (Fo)) -> Sum all Units (F0)/2
  Length (L0)/1 -> Fpe2/1, V,L/2
  Velocity (L0/s)/1 -> V,L/1
  Fpe2/1 -> Min/1
  zero2/1 -> Min/2
  Frequencies (f0.5)/1 -> Demux all Units/1
  Convert F0 to N/1 -> Force>0/1
  zero/1 -> Force>0/2
  Force>0/1 -> Force (N)/1
  Fpe1/1 -> Sum Forces (F0)/1
  Sum all Units (F0)/1 -> Sum Forces (F0)/2
  Sum Forces (F0)/1 -> Convert F0 to N/1

== system FinalSim/Shoulder Abductor/muscle mass ==
  Fce (N) : Inport
  Fse (N) : Inport  Port=2
  Path length [for init] (cm) : Inport  Port=3
  Acc to Vel : Integrator
  Force/Mass=Accel : Gain  Gain=1/0.02255  SaturateOnIntegerOverflow=on  OutDataTypeStr=Inherit: Same as input  ParamDataTypeStr=Inherit: Same as input
  Ftotal : Sum  Inputs=-+  InputSameDT=on  SaturateOnIntegerOverflow=on  OutDataTypeStr=Inherit: Same as first input
  Normalize to L0 : Gain  Gain=1/0.044  SaturateOnIntegerOverflow=on  OutDataTypeStr=Inherit: Same as input  ParamDataTypeStr=Inherit: Same as input
  Normalize to L0/s : Gain  Gain=1/0.044  SaturateOnIntegerOverflow=on  OutDataTypeStr=Inherit: Same as input  ParamDataTypeStr=Inherit: Same as input
  Path to init muscle mass position (m) : Fcn  Expr=(u-1.1106)/102.1232
  Vel to Pos : Integrator  InitialConditionSource=external
  Vce (L0/s) : Outport
  Lce (L0) : Outport  Port=2
  wires:
  Ftotal/1 -> Force/Mass=Accel/1
  Force/Mass=Accel/1 -> Acc to Vel/1
  Acc to Vel/1 -> Vel to Pos/1, Normalize to L0/s/1
  Path length [for init] (cm)/1 -> Path to init muscle mass position (m)/1
  Path to init muscle mass position (m)/1 -> Vel to Pos/2
  Vel to Pos/1 -> Normalize to L0/1
  Fce (N)/1 -> Ftotal/1
  Normalize to L0/1 -> Lce (L0)/1
  Fse (N)/1 -> Ftotal/2
  Normalize to L0/s/1 -> Vce (L0/s)/1

== system FinalSim/Shoulder Abductor/series elastic element ==
  Path (cm) : Inport
  Lce (L0) : Inport  Port=2
  Convert Lce to Lse : Sum  Inputs=+-  InputSameDT=on  SaturateOnIntegerOverflow=on  OutDataTypeStr=Inherit: Same as first input
  Convert to N : Gain  Gain=307.5  SaturateOnIntegerOverflow=on  OutDataTypeStr=Inherit: Same as input  ParamDataTypeStr=Inherit: Same as input
  Convert to cm : Gain  Gain=4.4  SaturateOnIntegerOverflow=on  OutDataTypeStr=Inherit: Same as input  ParamDataTypeStr=Inherit: Same as input
  Fse : Fcn  Expr=27.8*0.0047*log(exp((u(1)-0.964)/0.0047)+1)
  Normalize to L0T : Gain  Gain=1/1.3  SaturateOnIntegerOverflow=on  OutDataTypeStr=Inherit: Same as input  ParamDataTypeStr=Inherit: Same as input
  Fse (N) : Outport
  wires:
  Fse/1 -> Convert to N/1
  Normalize to L0T/1 -> Fse/1
  Convert Lce to Lse/1 -> Normalize to L0T/1
  Convert to N/1 -> Fse (N)/1
  Lce (L0)/1 -> Convert to cm/1
  Convert to cm/1 -> Convert Lce to Lse/2
  Path (cm)/1 -> Convert Lce to Lse/1

== system FinalSim/Shoulder Abductor Model/Shoulder Abductors1 ==
  Activation : Inport
  MT path length (m) : Inport  Port=2
  Convert m to cm : Gain  Gain=100  SaturateOnIntegerOverflow=on  OutDataTypeStr=Inherit: Same as input  ParamDataTypeStr=Inherit: Same as input
  Recruitment : Subsystem
  fascicles (CE & PE) : Subsystem
  muscle mass : Subsystem
  series elastic element : Subsystem
  Force (N) : Outport
  wires:
  MT path length (m)/1 -> Convert m to cm/1
  series elastic element/1(Fse (N)) -> muscle mass/2(Fse (N)), Force (N)/1
  fascicles (CE & PE)/1(Force (N)) -> muscle mass/1(Fce (N))
  muscle mass/2(Lce (L0)) -> series elastic element/2(Lce (L0)), fascicles (CE & PE)/2(Length (L0))
  muscle mass/1(Vce (L0/s)) -> fascicles (CE & PE)/3(Velocity (L0/s))
  Recruitment/1(Frequencies (f0.5)) -> fascicles (CE & PE)/1(Frequencies (f0.5))
  Convert m to cm/1 -> series elastic element/1(Path (cm)), muscle mass/3(Path length [for init] (cm))
  Activation/1 -> Recruitment/1(Activation)

== system FinalSim/Shoulder Adductor/Recruitment ==
  Activation : Inport
  Mux all F Units : Mux  Inputs=3
  Mux all S Units : Mux  Inputs=2
  Mux all Units : Mux  Inputs=2
  Type F Motor Unit 1 : Subsystem
  Type F Motor Unit 2 : Subsystem
  Type F Motor Unit 3 : Subsystem
  Type S Motor Unit 1 : Subsystem
  Type S Motor Unit 2 : Subsystem
  Frequencies (f0.5) : Outport
  wires:
  Activation/1 -> Type S Motor Unit 1/1(Activation), Type S Motor Unit 2/1(Activation), Type F Motor Unit 1/1(Activation), Type F Motor Unit 2/1(Activation), Type F Motor Unit 3/1(Activation)
  Type S Motor Unit 1/1(Frequency (f0.5)) -> Mux all S Units/1
  Type S Motor Unit 2/1(Frequency (f0.5)) -> Mux all S Units/2
  Mux all S Units/1 -> Mux all Units/1
  Type F Motor Unit 1/1(Frequency (f0.5)) -> Mux all F Units/1
  Type F Motor Unit 2/1(Frequency (f0.5)) -> Mux all F Units/2
  Type F Motor Unit 3/1(Frequency (f0.5)) -> Mux all F Units/3
  Mux all F Units/1 -> Mux all Units/2
  Mux all Units/1 -> Frequencies (f0.5)/1

== system FinalSim/Shoulder Adductor/fascicles (CE & PE) ==
  Frequencies (f0.5) : Inport
  Length (L0) : Inport  Port=2
  Velocity (L0/s) : Inport  Port=3
  Convert F0 to N : Gain  Gain=234.7059  SaturateOnIntegerOverflow=on  OutDataTypeStr=Inherit: Same as input  ParamDataTypeStr=Inherit: Same as input
  Demux all Units : Demux  Outputs="[2  3]"
      settings: DisplayOption=none
  Force>0 : MinMax  Function=max  Inputs=2  InputSameDT=on  SaturateOnIntegerOverflow=on
  Fpe1 : Fcn  Expr=0.01*u(1)+23*0.046*log(exp((u(2)/1.2845-1.17)/0.046)+1)
  Fpe2 : Fcn  Expr=-0.02*(exp(-21.0375*(u-0.70222))-1)
  Min : MinMax  Inputs=2  InputSameDT=on  SaturateOnIntegerOverflow=on
  Sum Forces (F0) : Sum  Inputs=2  InputSameDT=on  SaturateOnIntegerOverflow=on  OutDataTypeStr=Inherit: Same as first input
  Sum all Units (F0) : Sum  InputSameDT=on  SaturateOnIntegerOverflow=on  OutDataTypeStr=Inherit: Same as first input
  Type F Motor Units : Subsystem
  Type S Motor Units : Subsystem
  V,L : Mux  Inputs=2
  zero : Constant  Value=0
  zero2 : Constant  Value=0
  Force (N) : Outport
  wires:
  Demux all Units/1 -> Type S Motor Units/1(fenv)
  V,L/1 -> Type S Motor Units/2(V,L), Type F Motor Units/2(V,L), Fpe1/1
  Min/1 -> Type S Motor Units/3(Fpe2), Type F Motor Units/3(Fpe2)
  Type S Motor Units/1(F (Fo)) -> Sum all Units (F0)/1
  Demux all Units/2 -> Type F Motor Units/1(fenv)
  Type F Motor Units/1(F (Fo)) -> Sum all Units (F0)/2
  Length (L0)/1 -> Fpe2/1, V,L/2
  Velocity (L0/s)/1 -> V,L/1
  Fpe2/1 -> Min/1
  zero2/1 -> Min/2
  Frequencies (f0.5)/1 -> Demux all Units/1
  Convert F0 to N/1 -> Force>0/1
  zero/1 -> Force>0/2
  Force>0/1 -> Force (N)/1
  Fpe1/1 -> Sum Forces (F0)/1
  Sum all Units (F0)/1 -> Sum Forces (F0)/2
  Sum Forces (F0)/1 -> Convert F0 to N/1

== system FinalSim/Shoulder Adductor/muscle mass ==
  Fce (N) : Inport
  Fse (N) : Inport  Port=2
  Path length [for init] (cm) : Inport  Port=3
  Acc to Vel : Integrator
  Force/Mass=Accel : Gain  Gain=1/0.0266  SaturateOnIntegerOverflow=on  OutDataTypeStr=Inherit: Same as input  ParamDataTypeStr=Inherit: Same as input
  Ftotal : Sum  Inputs=-+  InputSameDT=on  SaturateOnIntegerOverflow=on  OutDataTypeStr=Inherit: Same as first input
  Normalize to L0 : Gain  Gain=1/0.068  SaturateOnIntegerOverflow=on  OutDataTypeStr=Inherit: Same as input  ParamDataTypeStr=Inherit: Same as input
  Normalize to L0/s : Gain  Gain=1/0.068  SaturateOnIntegerOverflow=on  OutDataTypeStr=Inherit: Same as input  ParamDataTypeStr=Inherit: Same as input
  Path to init muscle mass position (m) : Fcn  Expr=(u-0.68343)/100.9358
  Vel to Pos : Integrator  InitialConditionSource=external
  Vce (L0/s) : Outport
  Lce (L0) : Outport  Port=2
  wires:
  Ftotal/1 -> Force/Mass=Accel/1
  Force/Mass=Accel/1 -> Acc to Vel/1
  Acc to Vel/1 -> Vel to Pos/1, Normalize to L0/s/1
  Path length [for init] (cm)/1 -> Path to init muscle mass position (m)/1
  Path to init muscle mass position (m)/1 -> Vel to Pos/2
  Vel to Pos/1 -> Normalize to L0/1
  Fce (N)/1 -> Ftotal/1
  Normalize to L0/1 -> Lce (L0)/1
  Fse (N)/1 -> Ftotal/2
  Normalize to L0/s/1 -> Vce (L0/s)/1

== system FinalSim/Shoulder Adductor/series elastic element ==
  Path (cm) : Inport
  Lce (L0) : Inport  Port=2
  Convert Lce to Lse : Sum  Inputs=+-  InputSameDT=on  SaturateOnIntegerOverflow=on  OutDataTypeStr=Inherit: Same as first input
  Convert to N : Gain  Gain=234.7059  SaturateOnIntegerOverflow=on  OutDataTypeStr=Inherit: Same as input  ParamDataTypeStr=Inherit: Same as input
  Convert to cm : Gain  Gain=6.8  SaturateOnIntegerOverflow=on  OutDataTypeStr=Inherit: Same as input  ParamDataTypeStr=Inherit: Same as input
  Fse : Fcn  Expr=27.8*0.0047*log(exp((u(1)-0.964)/0.0047)+1)
  Normalize to L0T : Gain  Gain=1/0.8  SaturateOnIntegerOverflow=on  OutDataTypeStr=Inherit: Same as input  ParamDataTypeStr=Inherit: Same as input
  Fse (N) : Outport
  wires:
  Fse/1 -> Convert to N/1
  Normalize to L0T/1 -> Fse/1
  Convert Lce to Lse/1 -> Normalize to L0T/1
  Convert to N/1 -> Fse (N)/1
  Lce (L0)/1 -> Convert to cm/1
  Convert to cm/1 -> Convert Lce to Lse/2
  Path (cm)/1 -> Convert Lce to Lse/1

== system FinalSim/Shoulder Adductor Model/Shoulder Transverse Flexors1 ==
  Activation : Inport
  MT path length (m) : Inport  Port=2
  Convert m to cm : Gain  Gain=100  SaturateOnIntegerOverflow=on  OutDataTypeStr=Inherit: Same as input  ParamDataTypeStr=Inherit: Same as input
  Recruitment : Subsystem
  fascicles (CE & PE) : Subsystem
  muscle mass : Subsystem
  series elastic element : Subsystem
  Force (N) : Outport
  wires:
  MT path length (m)/1 -> Convert m to cm/1
  series elastic element/1(Fse (N)) -> muscle mass/2(Fse (N)), Force (N)/1
  fascicles (CE & PE)/1(Force (N)) -> muscle mass/1(Fce (N))
  muscle mass/2(Lce (L0)) -> series elastic element/2(Lce (L0)), fascicles (CE & PE)/2(Length (L0))
  muscle mass/1(Vce (L0/s)) -> fascicles (CE & PE)/3(Velocity (L0/s))
  Recruitment/1(Frequencies (f0.5)) -> fascicles (CE & PE)/1(Frequencies (f0.5))
  Convert m to cm/1 -> series elastic element/1(Path (cm)), muscle mass/3(Path length [for init] (cm))
  Activation/1 -> Recruitment/1(Activation)

== system FinalSim/Shoulder Extensor/Recruitment ==
  Activation : Inport
  Mux all F Units : Mux  Inputs=3
  Mux all S Units : Mux  Inputs=2
  Mux all Units : Mux  Inputs=2
  Type F Motor Unit 1 : Subsystem
  Type F Motor Unit 2 : Subsystem
  Type F Motor Unit 3 : Subsystem
  Type S Motor Unit 1 : Subsystem
  Type S Motor Unit 2 : Subsystem
  Frequencies (f0.5) : Outport
  wires:
  Activation/1 -> Type S Motor Unit 1/1(Activation), Type S Motor Unit 2/1(Activation), Type F Motor Unit 1/1(Activation), Type F Motor Unit 2/1(Activation), Type F Motor Unit 3/1(Activation)
  Type S Motor Unit 1/1(Frequency (f0.5)) -> Mux all S Units/1
  Type S Motor Unit 2/1(Frequency (f0.5)) -> Mux all S Units/2
  Mux all S Units/1 -> Mux all Units/1
  Type F Motor Unit 1/1(Frequency (f0.5)) -> Mux all F Units/1
  Type F Motor Unit 2/1(Frequency (f0.5)) -> Mux all F Units/2
  Type F Motor Unit 3/1(Frequency (f0.5)) -> Mux all F Units/3
  Mux all F Units/1 -> Mux all Units/2
  Mux all Units/1 -> Frequencies (f0.5)/1

== system FinalSim/Shoulder Extensor/fascicles (CE & PE) ==
  Frequencies (f0.5) : Inport
  Length (L0) : Inport  Port=2
  Velocity (L0/s) : Inport  Port=3
  Convert F0 to N : Gain  Gain=307.5  SaturateOnIntegerOverflow=on  OutDataTypeStr=Inherit: Same as input  ParamDataTypeStr=Inherit: Same as input
  Demux all Units : Demux  Outputs="[2  3]"
      settings: DisplayOption=none
  Force>0 : MinMax  Function=max  Inputs=2  InputSameDT=on  SaturateOnIntegerOverflow=on
  Fpe1 : Fcn  Expr=0.01*u(1)+23*0.046*log(exp((u(2)/1.4218-1.17)/0.046)+1)
  Fpe2 : Fcn  Expr=-0.02*(exp(-21.0375*(u-0.70222))-1)
  Min : MinMax  Inputs=2  InputSameDT=on  SaturateOnIntegerOverflow=on
  Sum Forces (F0) : Sum  Inputs=2  InputSameDT=on  SaturateOnIntegerOverflow=on  OutDataTypeStr=Inherit: Same as first input
  Sum all Units (F0) : Sum  InputSameDT=on  SaturateOnIntegerOverflow=on  OutDataTypeStr=Inherit: Same as first input
  Type F Motor Units : Subsystem
  Type S Motor Units : Subsystem
  V,L : Mux  Inputs=2
  zero : Constant  Value=0
  zero2 : Constant  Value=0
  Force (N) : Outport
  wires:
  Demux all Units/1 -> Type S Motor Units/1(fenv)
  V,L/1 -> Type S Motor Units/2(V,L), Type F Motor Units/2(V,L), Fpe1/1
  Min/1 -> Type S Motor Units/3(Fpe2), Type F Motor Units/3(Fpe2)
  Type S Motor Units/1(F (Fo)) -> Sum all Units (F0)/1
  Demux all Units/2 -> Type F Motor Units/1(fenv)
  Type F Motor Units/1(F (Fo)) -> Sum all Units (F0)/2
  Length (L0)/1 -> Fpe2/1, V,L/2
  Velocity (L0/s)/1 -> V,L/1
  Fpe2/1 -> Min/1
  zero2/1 -> Min/2
  Frequencies (f0.5)/1 -> Demux all Units/1
  Convert F0 to N/1 -> Force>0/1
  zero/1 -> Force>0/2
  Force>0/1 -> Force (N)/1
  Fpe1/1 -> Sum Forces (F0)/1
  Sum all Units (F0)/1 -> Sum Forces (F0)/2
  Sum Forces (F0)/1 -> Convert F0 to N/1

== system FinalSim/Shoulder Extensor/muscle mass ==
  Fce (N) : Inport
  Fse (N) : Inport  Port=2
  Path length [for init] (cm) : Inport  Port=3
  Acc to Vel : Integrator
  Force/Mass=Accel : Gain  Gain=1/0.02255  SaturateOnIntegerOverflow=on  OutDataTypeStr=Inherit: Same as input  ParamDataTypeStr=Inherit: Same as input
  Ftotal : Sum  Inputs=-+  InputSameDT=on  SaturateOnIntegerOverflow=on  OutDataTypeStr=Inherit: Same as first input
  Normalize to L0 : Gain  Gain=1/0.044  SaturateOnIntegerOverflow=on  OutDataTypeStr=Inherit: Same as input  ParamDataTypeStr=Inherit: Same as input
  Normalize to L0/s : Gain  Gain=1/0.044  SaturateOnIntegerOverflow=on  OutDataTypeStr=Inherit: Same as input  ParamDataTypeStr=Inherit: Same as input
  Path to init muscle mass position (m) : Fcn  Expr=(u-1.1106)/102.1232
  Vel to Pos : Integrator  InitialConditionSource=external
  Vce (L0/s) : Outport
  Lce (L0) : Outport  Port=2
  wires:
  Ftotal/1 -> Force/Mass=Accel/1
  Force/Mass=Accel/1 -> Acc to Vel/1
  Acc to Vel/1 -> Vel to Pos/1, Normalize to L0/s/1
  Path length [for init] (cm)/1 -> Path to init muscle mass position (m)/1
  Path to init muscle mass position (m)/1 -> Vel to Pos/2
  Vel to Pos/1 -> Normalize to L0/1
  Fce (N)/1 -> Ftotal/1
  Normalize to L0/1 -> Lce (L0)/1
  Fse (N)/1 -> Ftotal/2
  Normalize to L0/s/1 -> Vce (L0/s)/1

== system FinalSim/Shoulder Extensor/series elastic element ==
  Path (cm) : Inport
  Lce (L0) : Inport  Port=2
  Convert Lce to Lse : Sum  Inputs=+-  InputSameDT=on  SaturateOnIntegerOverflow=on  OutDataTypeStr=Inherit: Same as first input
  Convert to N : Gain  Gain=307.5  SaturateOnIntegerOverflow=on  OutDataTypeStr=Inherit: Same as input  ParamDataTypeStr=Inherit: Same as input
  Convert to cm : Gain  Gain=4.4  SaturateOnIntegerOverflow=on  OutDataTypeStr=Inherit: Same as input  ParamDataTypeStr=Inherit: Same as input
  Fse : Fcn  Expr=27.8*0.0047*log(exp((u(1)-0.964)/0.0047)+1)
  Normalize to L0T : Gain  Gain=1/1.3  SaturateOnIntegerOverflow=on  OutDataTypeStr=Inherit: Same as input  ParamDataTypeStr=Inherit: Same as input
  Fse (N) : Outport
  wires:
  Fse/1 -> Convert to N/1
  Normalize to L0T/1 -> Fse/1
  Convert Lce to Lse/1 -> Normalize to L0T/1
  Convert to N/1 -> Fse (N)/1
  Lce (L0)/1 -> Convert to cm/1
  Convert to cm/1 -> Convert Lce to Lse/2
  Path (cm)/1 -> Convert Lce to Lse/1

== system FinalSim/Shoulder Extensor Model/Shoulder Abductors1 ==
  Activation : Inport
  MT path length (m) : Inport  Port=2
  Convert m to cm : Gain  Gain=100  SaturateOnIntegerOverflow=on  OutDataTypeStr=Inherit: Same as input  ParamDataTypeStr=Inherit: Same as input
  Recruitment : Subsystem
  fascicles (CE & PE) : Subsystem
  muscle mass : Subsystem
  series elastic element : Subsystem
  Force (N) : Outport
  wires:
  MT path length (m)/1 -> Convert m to cm/1
  series elastic element/1(Fse (N)) -> muscle mass/2(Fse (N)), Force (N)/1
  fascicles (CE & PE)/1(Force (N)) -> muscle mass/1(Fce (N))
  muscle mass/2(Lce (L0)) -> series elastic element/2(Lce (L0)), fascicles (CE & PE)/2(Length (L0))
  muscle mass/1(Vce (L0/s)) -> fascicles (CE & PE)/3(Velocity (L0/s))
  Recruitment/1(Frequencies (f0.5)) -> fascicles (CE & PE)/1(Frequencies (f0.5))
  Convert m to cm/1 -> series elastic element/1(Path (cm)), muscle mass/3(Path length [for init] (cm))
  Activation/1 -> Recruitment/1(Activation)
